simulink model "blockdemo"  (Simulink 7.0)
settings: Solver=FixedStepDiscrete  StartTime=0.0  StopTime=10.0  FixedStep=1  RelTol=1e-3
InitFcn:
  | %% DSPBuilder Start
  | alt_dspbuilder_update_model(bdroot)
  | %% DSPBuilder End
libraries: allblocks_alteradspbuilder2 x21
settings Model: Creator=mjervis  LastModifiedBy=delphick
settings OptimizationCC: BooleanDataType=off  InlineInvariantSignals=on
settings DebuggingCC: SaveWithParameterizedLinksMsg=none  SignalResolutionControl=TryResolveAllWithWarning  SolverPrmCheckMsg=none  MultiTaskDSMMsg=warning  MultiTaskCondExecSysMsg=none
settings HardwareCC: TargetUnknown=on
settings RTWCC: IncludeERTFirstTime=on
settings GRTTargetCC: TargetFcnLib=ansi_tfl_tmw.mat

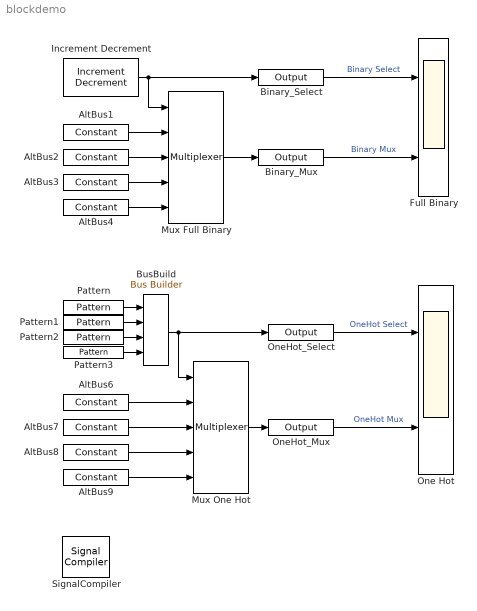
== system blockdemo ==
  AltBus1 : allblocks_alteradspbuilder2/Constant  mask_cst=1  BusType=Signed Integer  bwl=8  bwr=0  roundMode=Truncate  satMode=Wrap  SpecifyClock=off  allowFloatingPointOverride=on  logOutputs=off  logFile=C:\perforce_workspace81\main\dsp_builder2\Documentation\DesignExamples\Tutorials\UnitBlocks\GateAndControl\Multiplexer\tb_blockdemo\blockdemo_AltBus1.fixedpointlog
  AltBus2 : allblocks_alteradspbuilder2/Constant  mask_cst=2  BusType=Signed Integer  bwl=10  bwr=0  roundMode=Truncate  satMode=Wrap  SpecifyClock=off  allowFloatingPointOverride=on  logOutputs=off  logFile=C:\perforce_workspace81\main\dsp_builder2\Documentation\DesignExamples\Tutorials\UnitBlocks\GateAndControl\Multiplexer\tb_blockdemo\blockdemo_AltBus2.fixedpointlog
  AltBus3 : allblocks_alteradspbuilder2/Constant  mask_cst=3  BusType=Signed Integer  bwl=10  bwr=0  roundMode=Truncate  satMode=Wrap  SpecifyClock=off  allowFloatingPointOverride=on  logOutputs=off  logFile=C:\perforce_workspace81\main\dsp_builder2\Documentation\DesignExamples\Tutorials\UnitBlocks\GateAndControl\Multiplexer\tb_blockdemo\blockdemo_AltBus3.fixedpointlog
  AltBus4 : allblocks_alteradspbuilder2/Constant  mask_cst=4  BusType=Signed Integer  bwl=10  bwr=0  roundMode=Truncate  satMode=Wrap  SpecifyClock=off  allowFloatingPointOverride=on  logOutputs=off  logFile=C:\perforce_workspace81\main\dsp_builder2\Documentation\DesignExamples\Tutorials\UnitBlocks\GateAndControl\Multiplexer\tb_blockdemo\blockdemo_AltBus4.fixedpointlog
  AltBus6 : allblocks_alteradspbuilder2/Constant  mask_cst=10  BusType=Signed Integer  bwl=8  bwr=0  roundMode=Truncate  satMode=Wrap  SpecifyClock=off  allowFloatingPointOverride=on  logOutputs=off  logFile=C:\perforce_workspace81\main\dsp_builder2\Documentation\DesignExamples\Tutorials\UnitBlocks\GateAndControl\Multiplexer\tb_blockdemo\blockdemo_AltBus6.fixedpointlog
  AltBus7 : allblocks_alteradspbuilder2/Constant  mask_cst=20  BusType=Signed Integer  bwl=10  bwr=0  roundMode=Truncate  satMode=Wrap  SpecifyClock=off  allowFloatingPointOverride=on  logOutputs=off  logFile=C:\perforce_workspace81\main\dsp_builder2\Documentation\DesignExamples\Tutorials\UnitBlocks\GateAndControl\Multiplexer\tb_blockdemo\blockdemo_AltBus7.fixedpointlog
  AltBus8 : allblocks_alteradspbuilder2/Constant  mask_cst=30  BusType=Signed Integer  bwl=10  bwr=0  roundMode=Truncate  satMode=Wrap  SpecifyClock=off  allowFloatingPointOverride=on  logOutputs=off  logFile=C:\perforce_workspace81\main\dsp_builder2\Documentation\DesignExamples\Tutorials\UnitBlocks\GateAndControl\Multiplexer\tb_blockdemo\blockdemo_AltBus8.fixedpointlog
  AltBus9 : allblocks_alteradspbuilder2/Constant  mask_cst=40  BusType=Signed Integer  bwl=10  bwr=0  roundMode=Truncate  satMode=Wrap  SpecifyClock=off  allowFloatingPointOverride=on  logOutputs=off  logFile=C:\perforce_workspace81\main\dsp_builder2\Documentation\DesignExamples\Tutorials\UnitBlocks\GateAndControl\Multiplexer\tb_blockdemo\blockdemo_AltBus9.fixedpointlog
  Binary_Mux : allblocks_alteradspbuilder2/Output  iofile=C:\perforce_workspace81\main\dsp_builder2\Documentation\DesignExamples\Tutorials\UnitBlocks\GateAndControl\Multiplexer\tb_blockdemo\blockdemo_Binary%5FMux.capture  BusType=Inferred  bwl=10  bwr=0  externalType=Inferred  PORTTYPE=Output  allowFloatingPointOverride=on  logOutputs=off
  Binary_Select : allblocks_alteradspbuilder2/Output  iofile=C:\perforce_workspace81\main\dsp_builder2\Documentation\DesignExamples\Tutorials\UnitBlocks\GateAndControl\Multiplexer\tb_blockdemo\blockdemo_Binary%5FSelect.capture  BusType=Inferred  bwl=8  bwr=0  externalType=Inferred  PORTTYPE=Output  allowFloatingPointOverride=on  logOutputs=off
  BusBuild : allblocks_alteradspbuilder2/Bus Builder  BusType=Unsigned Integer  bwl=4  bwr=0  pipeline_display=0
  Full Binary : Scope  NumInputPorts=2
      settings: YMin=-2~-5  YMax=10~5
  Increment Decrement : allblocks_alteradspbuilder2/Increment Decrement  BusType=Unsigned Integer  bwl=4  bwr=0  SpecifyClock=off  clr_value=0  direction=Increment  phase_selection=1  use_ena=off  use_sclr=off  pipeline_display=1
  Mux Full Binary : allblocks_alteradspbuilder2/Multiplexer  numInputs=4  pipeline=0  oneHot=off  pipeline_display=0  use_ena=off  use_aclr=off  allowFloatingPointOverride=on  logOutputs=off  logFile=C:\perforce_workspace81\main\dsp_builder2\Documentation\DesignExamples\Tutorials\UnitBlocks\GateAndControl\Multiplexer\tb_blockdemo\blockdemo_Mux%0AFull+Binary.fixedpointlog
  Mux One Hot : allblocks_alteradspbuilder2/Multiplexer  numInputs=4  pipeline=0  oneHot=on  pipeline_display=0  use_ena=off  use_aclr=off  allowFloatingPointOverride=on  logOutputs=off  logFile=C:\perforce_workspace81\main\dsp_builder2\Documentation\DesignExamples\Tutorials\UnitBlocks\GateAndControl\Multiplexer\tb_blockdemo\blockdemo_Mux%0AOne+Hot.fixedpointlog
  One Hot : Scope  NumInputPorts=2
      settings: TickLabels=on  YMin=-2~0  YMax=10~45
  OneHot_Mux : allblocks_alteradspbuilder2/Output  iofile=C:\perforce_workspace81\main\dsp_builder2\Documentation\DesignExamples\Tutorials\UnitBlocks\GateAndControl\Multiplexer\tb_blockdemo\blockdemo_OneHot%5FMux.capture  BusType=Inferred  bwl=10  bwr=0  externalType=Inferred  PORTTYPE=Output  allowFloatingPointOverride=on  logOutputs=off
  OneHot_Select : allblocks_alteradspbuilder2/Output  iofile=C:\perforce_workspace81\main\dsp_builder2\Documentation\DesignExamples\Tutorials\UnitBlocks\GateAndControl\Multiplexer\tb_blockdemo\blockdemo_OneHot%5FSelect.capture  BusType=Inferred  bwl=4  bwr=0  externalType=Inferred  PORTTYPE=Output  allowFloatingPointOverride=on  logOutputs=off
  Pattern : allblocks_alteradspbuilder2/Pattern  Sequence=1000  SpecifyClock=off  use_ena=off  use_sclr=off
  Pattern1 : allblocks_alteradspbuilder2/Pattern  Sequence=0100  SpecifyClock=off  use_ena=off  use_sclr=off
  Pattern2 : allblocks_alteradspbuilder2/Pattern  Sequence=0010  SpecifyClock=off  use_ena=off  use_sclr=off
  Pattern3 : allblocks_alteradspbuilder2/Pattern  Sequence=0001  SpecifyClock=off  use_ena=off  use_sclr=off
  SignalCompiler : allblocks_alteradspbuilder2/Signal Compiler  DeviceFamily=Stratix IV  DeviceName=AUTO  EnableSignalTap=off  SignalTapDepth=128  UseBoardBlock=off  StpUseDefaultClock=on  StpClock=Clock  ExportDir=C:\Documents and Settings\delphick\My Documents\MATLAB
  wires:
  Mux Full Binary/1 -> Binary_Mux/1
  Increment Decrement/1 -> Mux Full Binary/1, Binary_Select/1
  AltBus1/1 -> Mux Full Binary/2
  AltBus2/1 -> Mux Full Binary/3
  AltBus3/1 -> Mux Full Binary/4
  AltBus4/1 -> Mux Full Binary/5
  Binary_Mux/1 -> Full Binary/2  "Binary Mux"
  Mux One Hot/1 -> OneHot_Mux/1
  BusBuild/1 -> Mux One Hot/1, OneHot_Select/1
  AltBus6/1 -> Mux One Hot/2
  AltBus7/1 -> Mux One Hot/3
  AltBus8/1 -> Mux One Hot/4
  AltBus9/1 -> Mux One Hot/5
  OneHot_Mux/1 -> One Hot/2  "OneHot Mux"
  Pattern/1 -> BusBuild/1
  Pattern1/1 -> BusBuild/2
  Pattern2/1 -> BusBuild/3
  Pattern3/1 -> BusBuild/4
  Binary_Select/1 -> Full Binary/1  "Binary Select"
  OneHot_Select/1 -> One Hot/1  "OneHot Select"
